simulink model "q3_model"  (R2016a)
settings: Solver=FixedStepAuto  StartTime=0.0  StopTime=25  FixedStep=1e-3  RelTol=1e-3
values from neighbouring files (symbols this model uses):
  A = double(subs(jacobian(f,x),[x1 x2 x3 x4],[0 0 0 0]))    [q3.m]    (also in q3_daniel.m)
  Am = M    (= 1)    [q3.m]
  Am_q5 = M_q5    [q3.m]
  B = double(subs(uf,[x3 x4],[0 0]))    [q3.m]    (also in q3_daniel.m)
  Bm = N    [q3.m]
  Bm_q5 = N_q5    [q3.m]
  C = [1 0 0 0]    [q3.m]    (also in q3_daniel.m)
  Cm = eye(1)    [q3.m]
  Cm_q5 = eye(3)    [q3.m]
  Dm = zeros(1,1)    [q3.m]
  Dm_q5 = zeros(3,1)    [q3.m]
  Dsim = zeros(4,1)    [q3.m]
  K = Ka(:,1:4)    [q3.m]    (also in q3_daniel.m = place(A,B, [pd pd-.01 pd+0.05 pd+0.02]))
  K_q5 = Ka_q5(:,1:4)    [q3.m]
  Km = Ka(5)    [q3.m]    (also in q3_daniel.m = Ka(1,5))
  Km_q5 = Ka_q5(5:7)    [q3.m]
  Kx_lqr = Ka_lqr(1,1:4)    [q3.m]
  L = H'    [q3.m]    (also in q3_daniel.m = 1)
  x0 = [0 0 pi/180*25 0]    [q3.m]    (also in q3_daniel.m = [0 0 pi/180*12 0])
  x0Obs = [0; 0; pi/180*10; 0]    [q3.m]
settings Model: Creator=ivan_prog  LastModifiedBy=ivan_prog

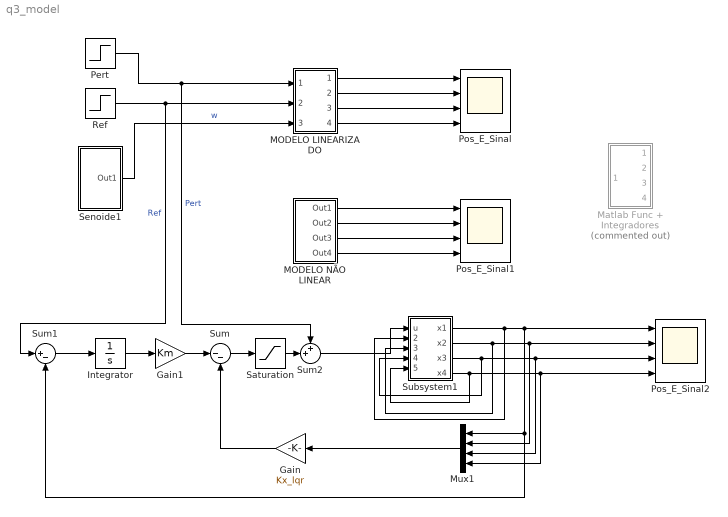
== system q3_model ==
  Gain : Gain  Gain=Kx_lqr
  Gain1 : Gain  Gain=Km
  Integrator : Integrator
  MODELO LINEARIZADO : Subsystem
  MODELO NÃO LINEAR : Subsystem
  Matlab Func + Integradores : Subsystem  Commented=on
  Mux1 : Mux
  Pert : Step  Time=10  After=-10  SampleTime=0
  Pos_E_Sinal : Scope  NumInputPorts=4
  Pos_E_Sinal1 : Scope  NumInputPorts=4
  Pos_E_Sinal2 : Scope  NumInputPorts=4
  Ref : Step  Time=0  After=5  SampleTime=0
  Saturation : Saturate  UpperLimit=50  LowerLimit=-50
  Senoide1 : Subsystem
  Subsystem1 : Subsystem
  Sum : Sum  Inputs=|--
  Sum1 : Sum  Inputs=|+-
  Sum2 : Sum  Inputs=++|
  wires:
  Pert/1 -> MODELO LINEARIZADO/1(In1), Sum2/1  "Pert"
  Ref/1 -> Sum1/1, MODELO LINEARIZADO/2(In2)  "Ref"
  Senoide1/1(Out1) -> MODELO LINEARIZADO/3(In3)  "w"
  MODELO LINEARIZADO/1(Out1) -> Pos_E_Sinal/1
  MODELO LINEARIZADO/2(Out2) -> Pos_E_Sinal/2
  MODELO LINEARIZADO/3(Out3) -> Pos_E_Sinal/3
  MODELO LINEARIZADO/4(Out4) -> Pos_E_Sinal/4
  MODELO NÃO LINEAR/1(Out1) -> Pos_E_Sinal1/1
  MODELO NÃO LINEAR/2(Out2) -> Pos_E_Sinal1/2
  MODELO NÃO LINEAR/3(Out3) -> Pos_E_Sinal1/3
  MODELO NÃO LINEAR/4(Out4) -> Pos_E_Sinal1/4
  Subsystem1/4(x4) -> Subsystem1/5(x4e), Pos_E_Sinal2/4, Mux1/4
  Subsystem1/3(x3) -> Subsystem1/4(x3e), Pos_E_Sinal2/3, Mux1/3
  Subsystem1/1(x1) -> Subsystem1/2(x1e), Pos_E_Sinal2/1, Sum1/2, Mux1/1
  Mux1/1 -> Gain/1
  Gain/1 -> Sum/2
  Sum/1 -> Saturation/1
  Gain1/1 -> Sum/1
  Integrator/1 -> Gain1/1
  Sum1/1 -> Integrator/1
  Saturation/1 -> Sum2/2
  Sum2/1 -> Subsystem1/1(u)
  Subsystem1/2(x2) -> Subsystem1/3(x2e), Pos_E_Sinal2/2, Mux1/2

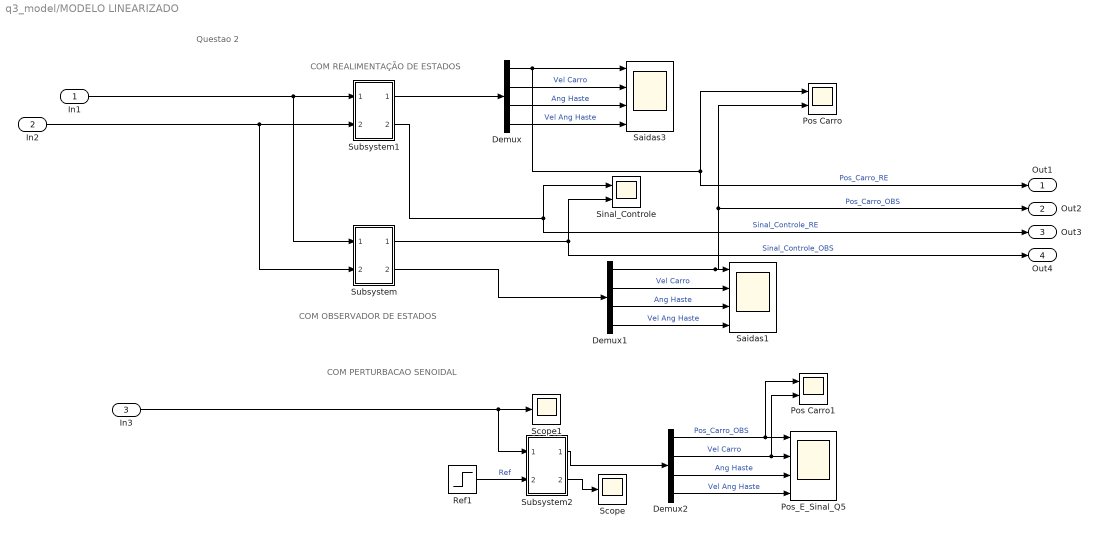
== system q3_model/MODELO LINEARIZADO ==
  note: Questao 2
  note: COM PERTURBACAO SENOIDAL
  note: COM OBSERVADOR DE ESTADOS
  note: COM REALIMENTAÇÃO DE ESTADOS
  In1 : Inport
  In2 : Inport  Port=2
  In3 : Inport  Port=3
  Demux : Demux
  Demux1 : Demux
  Demux2 : Demux
  Pos Carro : Scope  NumInputPorts=2
  Pos Carro1 : Scope  NumInputPorts=2
  Pos_E_Sinal_Q5 : Scope  NumInputPorts=4
  Ref1 : Step  Time=0  After=0  SampleTime=0
  Saidas1 : Scope  NumInputPorts=4
  Saidas3 : Scope  NumInputPorts=4
  Scope : Scope
  Scope1 : Scope
  Sinal_Controle : Scope  NumInputPorts=2
  Subsystem : Subsystem
  Subsystem1 : Subsystem
  Subsystem2 : Subsystem
  Out1 : Outport
  Out2 : Outport  Port=2
  Out3 : Outport  Port=3
  Out4 : Outport  Port=4
  wires:
  Subsystem2/1(Out1) -> Demux2/1
  Demux1/4 -> Saidas1/4  "Vel Ang Haste"
  Demux2/1 -> Pos Carro1/1, Pos_E_Sinal_Q5/1  "Pos_Carro_OBS"
  Demux/1 -> Saidas3/1, Out1/1, Pos Carro/1  "Pos_Carro_RE"
  Demux/2 -> Saidas3/2  "Vel Carro"
  Ref1/1 -> Subsystem2/2(In2)  "Ref"
  Subsystem1/2(Out2) -> Out3/1, Sinal_Controle/1  "Sinal_Controle_RE"
  Demux2/4 -> Pos_E_Sinal_Q5/4  "Vel Ang Haste"
  Subsystem/1(Out1) -> Out4/1, Sinal_Controle/2  "Sinal_Controle_OBS"
  Subsystem/2(Out2) -> Demux1/1
  Demux1/3 -> Saidas1/3  "Ang Haste"
  Demux1/1 -> Out2/1, Pos Carro/2, Saidas1/1  "Pos_Carro_OBS"
  Demux2/2 -> Pos Carro1/2, Pos_E_Sinal_Q5/2  "Vel Carro"
  Subsystem1/1(Out1) -> Demux/1
  In2/1 -> Subsystem/2(In2), Subsystem1/2(In2)
  Demux2/3 -> Pos_E_Sinal_Q5/3  "Ang Haste"
  Demux1/2 -> Saidas1/2  "Vel Carro"
  Demux/4 -> Saidas3/4  "Vel Ang Haste"
  Demux/3 -> Saidas3/3  "Ang Haste"
  In3/1 -> Scope1/1, Subsystem2/1(In1)
  Subsystem2/2(Out2) -> Scope/1
  In1/1 -> Subsystem/1(In1), Subsystem1/1(In1)

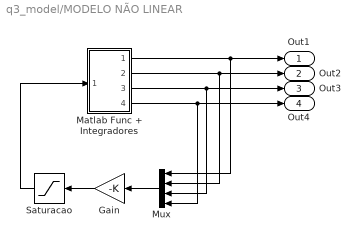
== system q3_model/MODELO NÃO LINEAR ==
  Gain : Gain  Gain=-K
  Matlab Func + Integradores : Subsystem
  Mux : Mux
  Saturacao : Saturate  UpperLimit=50  LowerLimit=-50
  Out1 : Outport
  Out2 : Outport  Port=2
  Out3 : Outport  Port=3
  Out4 : Outport  Port=4
  wires:
  Matlab Func + Integradores/1(Out1) -> Out1/1, Mux/1
  Matlab Func + Integradores/3(Out3) -> Out3/1, Mux/3
  Matlab Func + Integradores/2(Out2) -> Out2/1, Mux/2
  Matlab Func + Integradores/4(Out4) -> Out4/1, Mux/4
  Mux/1 -> Gain/1
  Gain/1 -> Saturacao/1
  Saturacao/1 -> Matlab Func + Integradores/1(In1)

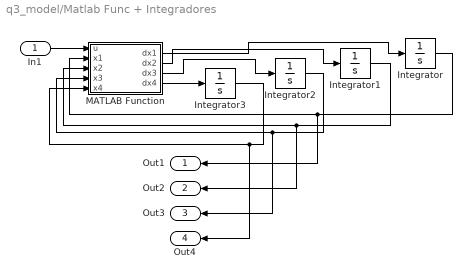
== system q3_model/Matlab Func + Integradores ==
  In1 : Inport
  Integrator{,1..3} (4 alike) : Integrator
  MATLAB Function : MATLAB Function  TreatAsAtomicUnit=on
  Out1 : Outport
  Out2 : Outport  Port=2
  Out3 : Outport  Port=3
  Out4 : Outport  Port=4
  wires:
  MATLAB Function/4(dx4) -> Integrator3/1
  Integrator/1 -> Out1/1, MATLAB Function/2(x1)
  Integrator1/1 -> Out2/1, MATLAB Function/3(x2)
  Integrator3/1 -> MATLAB Function/5(x4), Out4/1
  Integrator2/1 -> MATLAB Function/4(x3), Out3/1
  In1/1 -> MATLAB Function/1(u)
  MATLAB Function/2(dx2) -> Integrator1/1
  MATLAB Function/1(dx1) -> Integrator/1
  MATLAB Function/3(dx3) -> Integrator2/1

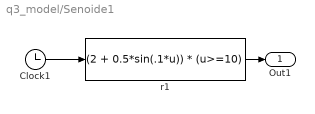
== system q3_model/Senoide1 ==
  Clock1 : Clock
  r1 : Fcn  Expr="(2 + 0.5*sin(.1*u))  * (u>=10)"
  Out1 : Outport
  wires:
  Clock1/1 -> r1/1
  r1/1 -> Out1/1

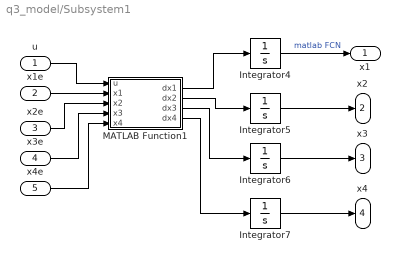
== system q3_model/Subsystem1 ==
  u : Inport
  x1e : Inport  Port=2
  x2e : Inport  Port=3
  x3e : Inport  Port=4
  x4e : Inport  Port=5
  Integrator4 : Integrator  InitialCondition=x0(1)  ZeroCross=off
  Integrator5 : Integrator  InitialCondition=x0(2)  ZeroCross=off
  Integrator6 : Integrator  InitialCondition=x0(3)  ZeroCross=off
  Integrator7 : Integrator  InitialCondition=x0(4)  ZeroCross=off
  MATLAB Function1 : MATLAB Function  TreatAsAtomicUnit=on
  x1 : Outport
  x2 : Outport  Port=2
  x3 : Outport  Port=3
  x4 : Outport  Port=4
  wires:
  Integrator6/1 -> x3/1
  MATLAB Function1/2(dx2) -> Integrator5/1
  MATLAB Function1/3(dx3) -> Integrator6/1
  Integrator4/1 -> x1/1  "matlab FCN"
  MATLAB Function1/1(dx1) -> Integrator4/1
  MATLAB Function1/4(dx4) -> Integrator7/1
  u/1 -> MATLAB Function1/1(u)
  Integrator7/1 -> x4/1
  Integrator5/1 -> x2/1
  x1e/1 -> MATLAB Function1/2(x1)
  x3e/1 -> MATLAB Function1/4(x3)
  x4e/1 -> MATLAB Function1/5(x4)
  x2e/1 -> MATLAB Function1/3(x2)

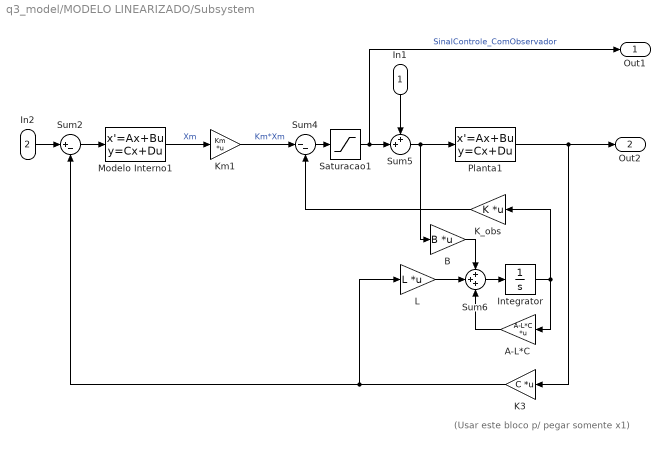
== system q3_model/MODELO LINEARIZADO/Subsystem ==
  note: (Usar este bloco p/ pegar somente x1)
  In1 : Inport
  In2 : Inport  Port=2
  A-L*C : Gain  Gain=A-L*C  Multiplication=Matrix(K*u)
  B : Gain  Gain=B  Multiplication=Matrix(K*u)
  Integrator : Integrator  InitialCondition=x0Obs
  K3 : Gain  Gain=C  Multiplication=Matrix(K*u)
  K_obs : Gain  Gain=K  Multiplication=Matrix(K*u)
  Km1 : Gain  Gain=Km  Multiplication=Matrix(K*u)
  L : Gain  Gain=L  Multiplication=Matrix(K*u)
  Modelo Interno1 : StateSpace  A=Am  B=Bm  C=Cm  D=Dm  X0=[0]
  Planta1 : StateSpace  A=A  B=B  C=eye(4)  D=Dsim  X0=x0
  Saturacao1 : Saturate  UpperLimit=50  LowerLimit=-50
  Sum2 : Sum  Inputs=|+-
  Sum4 : Sum  Inputs=|--
  Sum5 : Sum  Inputs=++|
  Sum6 : Sum  Inputs=+++
  Out1 : Outport
  Out2 : Outport  Port=2
  wires:
  A-L*C/1 -> Sum6/3
  Sum5/1 -> Planta1/1, B/1
  B/1 -> Sum6/1
  Sum2/1 -> Modelo Interno1/1
  L/1 -> Sum6/2
  K3/1 -> L/1, Sum2/2
  Planta1/1 -> Out2/1, K3/1
  In2/1 -> Sum2/1
  In1/1 -> Sum5/1
  Sum4/1 -> Saturacao1/1
  Saturacao1/1 -> Sum5/2, Out1/1  "SinalControle_ComObservador"
  Km1/1 -> Sum4/1  "Km*Xm"
  Modelo Interno1/1 -> Km1/1  "Xm"
  Integrator/1 -> K_obs/1, A-L*C/1
  Sum6/1 -> Integrator/1
  K_obs/1 -> Sum4/2

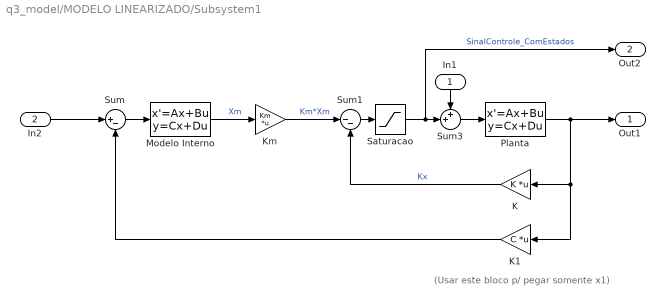
== system q3_model/MODELO LINEARIZADO/Subsystem1 ==
  note: (Usar este bloco p/ pegar somente x1)
  In1 : Inport
  In2 : Inport  Port=2
  K : Gain  Gain=K  Multiplication=Matrix(K*u)
  K1 : Gain  Gain=C  Multiplication=Matrix(K*u)
  Km : Gain  Gain=Km  Multiplication=Matrix(K*u)
  Modelo Interno : StateSpace  A=Am  B=Bm  C=Cm  D=Dm  X0=[0]
  Planta : StateSpace  A=A  B=B  C=eye(4)  D=Dsim  X0=x0
  Saturacao : Saturate  UpperLimit=50  LowerLimit=-50
  Sum : Sum  Inputs=|+-
  Sum1 : Sum  Inputs=|--
  Sum3 : Sum  Inputs=++|
  Out1 : Outport
  Out2 : Outport  Port=2
  wires:
  Km/1 -> Sum1/1  "Km*Xm"
  Modelo Interno/1 -> Km/1  "Xm"
  Sum3/1 -> Planta/1
  K/1 -> Sum1/2  "Kx"
  In1/1 -> Sum3/1
  In2/1 -> Sum/1
  Sum/1 -> Modelo Interno/1
  Planta/1 -> Out1/1, K1/1, K/1
  Saturacao/1 -> Out2/1, Sum3/2  "SinalControle_ComEstados"
  Sum1/1 -> Saturacao/1
  K1/1 -> Sum/2

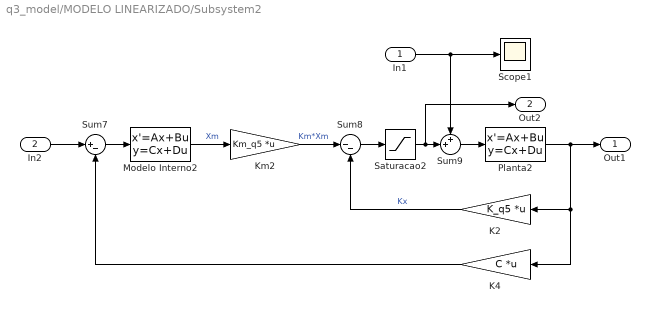
== system q3_model/MODELO LINEARIZADO/Subsystem2 ==
  In1 : Inport
  In2 : Inport  Port=2
  K2 : Gain  Gain=K_q5  Multiplication=Matrix(K*u)
  K4 : Gain  Gain=C  Multiplication=Matrix(K*u)
  Km2 : Gain  Gain=Km_q5  Multiplication=Matrix(K*u)
  Modelo Interno2 : StateSpace  A=Am_q5  B=Bm_q5  C=Cm_q5  D=Dm_q5  X0=[0]
  Planta2 : StateSpace  A=A  B=B  C=eye(4)  D=Dsim  X0=x0
  Saturacao2 : Saturate  UpperLimit=50  LowerLimit=-50
  Scope1 : Scope
  Sum7 : Sum  Inputs=|+-
  Sum8 : Sum  Inputs=|--
  Sum9 : Sum  Inputs=++|
  Out1 : Outport
  Out2 : Outport  Port=2
  wires:
  Km2/1 -> Sum8/1  "Km*Xm"
  Sum9/1 -> Planta2/1
  K4/1 -> Sum7/2
  Sum7/1 -> Modelo Interno2/1
  K2/1 -> Sum8/2  "Kx"
  Sum8/1 -> Saturacao2/1
  Modelo Interno2/1 -> Km2/1  "Xm"
  In1/1 -> Scope1/1, Sum9/1
  In2/1 -> Sum7/1
  Planta2/1 -> Out1/1, K2/1, K4/1
  Saturacao2/1 -> Out2/1, Sum9/2

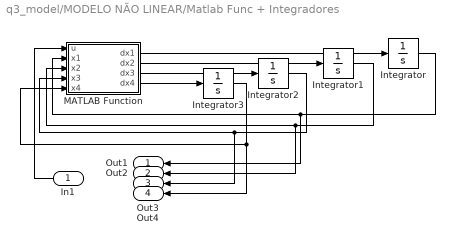
== system q3_model/MODELO NÃO LINEAR/Matlab Func + Integradores ==
  In1 : Inport
  Integrator{,1..3} (4 alike) : Integrator
  MATLAB Function : MATLAB Function  TreatAsAtomicUnit=on
  Out1 : Outport
  Out2 : Outport  Port=2
  Out3 : Outport  Port=3
  Out4 : Outport  Port=4
  wires:
  MATLAB Function/4(dx4) -> Integrator3/1
  Integrator/1 -> Out1/1, MATLAB Function/2(x1)
  Integrator1/1 -> Out2/1, MATLAB Function/3(x2)
  Integrator3/1 -> Out4/1, MATLAB Function/5(x4)
  Integrator2/1 -> Out3/1, MATLAB Function/4(x3)
  In1/1 -> MATLAB Function/1(u)
  MATLAB Function/2(dx2) -> Integrator1/1
  MATLAB Function/1(dx1) -> Integrator/1
  MATLAB Function/3(dx3) -> Integrator2/1

== matlab function q3_model/Matlab Func + Integradores/MATLAB Function ==
  data: u input; dx1 output; x1 input; x2 input; x3 input; x4 input; dx2 output; dx3 output; dx4 output
function [dx1,dx2,dx3,dx4] = fcn(u, x1, x2, x3, x4)
%#codegen
M = 1;
L = 1;
m = 0.5;
g = 9.81;


dx1 = x2;
dx2 = (u-m*g*sin(x3)*cos(x3)+m*L*x4^2*sin(x3))/(M+m-m*cos(x3)^2);
dx3 = x4;
f4_num = m*g*sin(x3)-((u+m*L*x4^2*sin(x3))*m*cos(x3))/(M+m);
f4_den = m*L-(m^2*L*cos(x3)^2)/(M+m);
dx4 = f4_num/f4_den;

end

== matlab function q3_model/MODELO NÃO LINEAR/Matlab Func + Integradores/MATLAB Function ==
  data: u input; dx1 output; x1 input; x2 input; x3 input; x4 input; dx2 output; dx3 output; dx4 output
function [dx1,dx2,dx3,dx4] = fcn(u, x1, x2, x3, x4)
%#codegen
M = 1;
L = 1;
m = 0.5;
g = 9.81;


dx1 = x2;
dx2 = (u-m*g*sin(x3)*cos(x3)+m*L*x4^2*sin(x3))/(M+m-m*cos(x3)^2);
dx3 = x4;
f4_num = m*g*sin(x3)-((u+m*L*x4^2*sin(x3))*m*cos(x3))/(M+m);
f4_den = m*L-(m^2*L*cos(x3)^2)/(M+m);
dx4 = f4_num/f4_den;

end

== matlab function q3_model/Subsystem1/MATLAB Function1 ==
  data: dx1 output; dx2 output; dx3 output; u input; x1 input; x2 input; x3 input; x4 input; dx4 output
function [dx1,dx2,dx3,dx4] = fcn(u, x1, x2, x3, x4)
%#codegen
M = 1;
L = 1;
m = 0.5;
g = 9.81;


dx1 = x2;
dx2 = (u-m*g*sin(x3)*cos(x3)+m*L*x4^2*sin(x3))/(M+m-m*cos(x3)^2);
dx3 = x4;
f4_num = m*g*sin(x3)-((u+m*L*x4^2*sin(x3))*m*cos(x3))/(M+m);
f4_den = m*L-(m^2*L*cos(x3)^2)/(M+m);
dx4 = f4_num/f4_den;

end
